simulink model "mpc_nonlinear_ss"  (Simulink 7.0)
settings: Solver=ode45  SolverMode=SingleTasking  StartTime=0.0  StopTime=Tfinal  RelTol=1e-3
values from neighbouring files (symbols this model uses):
  refs = [1;1]    [mpcnonlinear.m]    (also in simmismatch.m = [1 2])
libraries: cstblocks x1, mpclib x1
settings Model: Creator=jowen  LastModifiedBy=rchen  ExtModeTrigMode=oneshot  ExtModeArmWhenConnect=off
settings DataIOCC: LimitDataPoints=off  SignalLoggingName=sigsOut
settings OptimizationCC: BooleanDataType=off  InlineInvariantSignals=on
settings DebuggingCC: CheckExecutionContextPreStartOutputMsg=on  CheckExecutionContextRuntimeOutputMsg=on  SignalResolutionControl=TryResolveAllWithWarning  SolverPrmCheckMsg=none  MultiTaskDSMMsg=warning  MultiTaskCondExecSysMsg=none  IntegerOverflowMsg=none  StrictBusMsg=None
settings HardwareCC: TargetUnknown=on
settings RTWCC: IncludeERTFirstTime=on

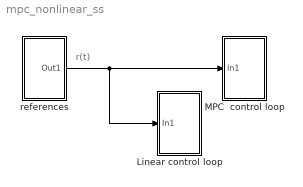
== system mpc_nonlinear_ss ==
  note: r(t)
  Linear control loop : Subsystem
  MPC  control loop : Subsystem
  references : Subsystem
  wires:
  references/1(Out1) -> MPC  control loop/1(In1), Linear control loop/1(In1)

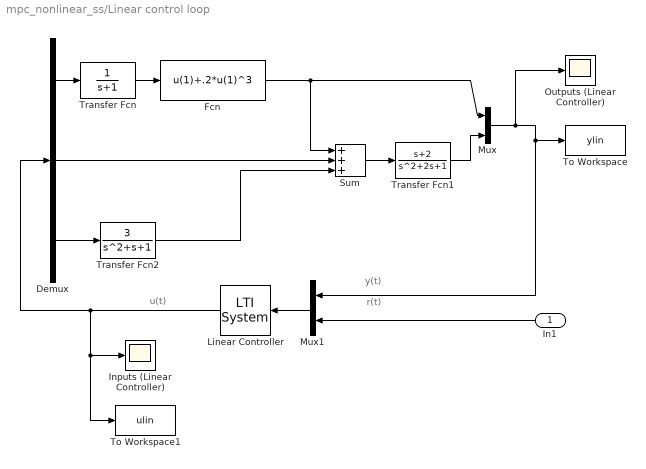
== system mpc_nonlinear_ss/Linear control loop ==
  note: r(t)
  note: y(t)
  note: u(t)
  In1 : Inport  Orientation=left
  Demux : Demux  Outputs=3
  Fcn : Fcn  Expr=u(1)+.2*u(1)^3
  Inputs (Linear Controller) : Scope
      settings: TimeRange=8  YMin=-2  YMax=2  DataFormat=Structure
  Linear Controller : cstblocks/LTI System  Orientation=left  sys=LTIMPC  IC=0
  Mux : Mux  Inputs=2
  Mux1 : Mux  Orientation=left  Inputs=2
  Outputs (Linear Controller) : Scope
      settings: TimeRange=8  YMin=-0.5  YMax=1.5  DataFormat=Structure
  Sum : Sum  Inputs=+++  SaturateOnIntegerOverflow=on  InputSameDT=on
  To Workspace : ToWorkspace  VariableName=ylin  SampleTime=-1  SaveFormat=Array
      settings: MaxDataPoints=Inf
  To Workspace1 : ToWorkspace  VariableName=ulin  SampleTime=-1  SaveFormat=Array
      settings: MaxDataPoints=Inf
  Transfer Fcn : TransferFcn  Denominator=[1 1]
  Transfer Fcn1 : TransferFcn  Numerator=[1 2]
  Transfer Fcn2 : TransferFcn  Numerator=[3]  Denominator=[1 1 1]
  wires:
  In1/1 -> Mux1/2
  Transfer Fcn1/1 -> Mux/2
  Demux/1 -> Transfer Fcn/1
  Sum/1 -> Transfer Fcn1/1
  Demux/2 -> Sum/2
  Fcn/1 -> Mux/1, Sum/1
  Transfer Fcn/1 -> Fcn/1
  Transfer Fcn2/1 -> Sum/3
  Demux/3 -> Transfer Fcn2/1
  Mux/1 -> To Workspace/1, Mux1/1, Outputs (Linear Controller)/1
  Linear Controller/1 -> Inputs (Linear Controller)/1, To Workspace1/1, Demux/1
  Mux1/1 -> Linear Controller/1

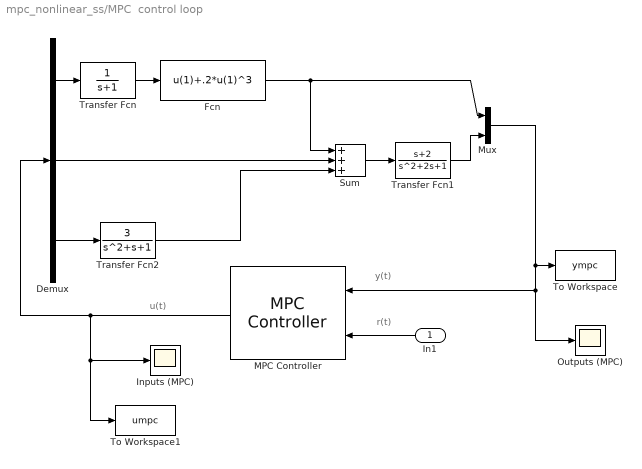
== system mpc_nonlinear_ss/MPC  control loop ==
  note: u(t)
  note: y(t)
  note: r(t)
  In1 : Inport  Orientation=left
  Demux : Demux  Outputs=3
  Fcn : Fcn  Expr=u(1)+.2*u(1)^3
  Inputs (MPC) : Scope
      settings: TimeRange=8  YMin=-2  YMax=2  DataFormat=Structure
  MPC Controller : mpclib/MPC Controller  Orientation=left  SystemSampleTime=-1  mpcobj=MPCobj  n_mv=0  x0=[]  ref_from_ws=off  ref_signal_name=[]  ref_preview=on  md_from_ws=off  md_signal_name=[]  md_preview=on  from_project=off  md_inport=off  mv_inport=off  lims_inport=off  project_file=MPCtask.mat
  Mux : Mux  Inputs=2
  Outputs (MPC) : Scope
      settings: TimeRange=8  YMin=-0.5  YMax=1.5  DataFormat=Structure
  Sum : Sum  Inputs=+++  SaturateOnIntegerOverflow=on  InputSameDT=on
  To Workspace : ToWorkspace  VariableName=ympc  SampleTime=-1  SaveFormat=Array
      settings: MaxDataPoints=Inf
  To Workspace1 : ToWorkspace  VariableName=umpc  SampleTime=-1  SaveFormat=Array
      settings: MaxDataPoints=Inf
  Transfer Fcn : TransferFcn  Denominator=[1 1]
  Transfer Fcn1 : TransferFcn  Numerator=[1 2]
  Transfer Fcn2 : TransferFcn  Numerator=[3]  Denominator=[1 1 1]
  wires:
  MPC Controller/1 -> Demux/1, To Workspace1/1, Inputs (MPC)/1
  Mux/1 -> Outputs (MPC)/1, MPC Controller/1, To Workspace/1
  Demux/3 -> Transfer Fcn2/1
  Transfer Fcn2/1 -> Sum/3
  Transfer Fcn/1 -> Fcn/1
  Fcn/1 -> Sum/1, Mux/1
  Demux/2 -> Sum/2
  Sum/1 -> Transfer Fcn1/1
  Demux/1 -> Transfer Fcn/1
  Transfer Fcn1/1 -> Mux/2
  In1/1 -> MPC Controller/2

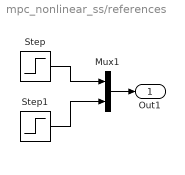
== system mpc_nonlinear_ss/references ==
  Mux1 : Mux  Inputs=2
  Step : Step  Time=4  Before=refs(1)  After=0  SampleTime=0
  Step1 : Step  Time=0  After=refs(2)  SampleTime=0
  Out1 : Outport
  wires:
  Step/1 -> Mux1/1
  Step1/1 -> Mux1/2
  Mux1/1 -> Out1/1
